simulink model "testing"  (R2023b)
settings: Solver=FixedStepAuto  StartTime=0.0  StopTime=2  FixedStep=0.001  MaxStep=0.02  RelTol=1e-3
undefined symbols (not defined in the file or in its folder): b_t, bt_eq, i_t, Jt_eq, m_t, r_td
libraries: robotcorelib x2
settings Model: Creator=Ferran  LastModifiedBy=Ferran

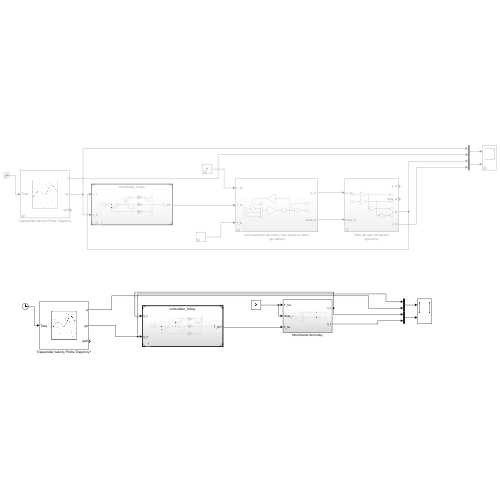
[thumbnail: Simulink's stored preview of the top-level diagram]
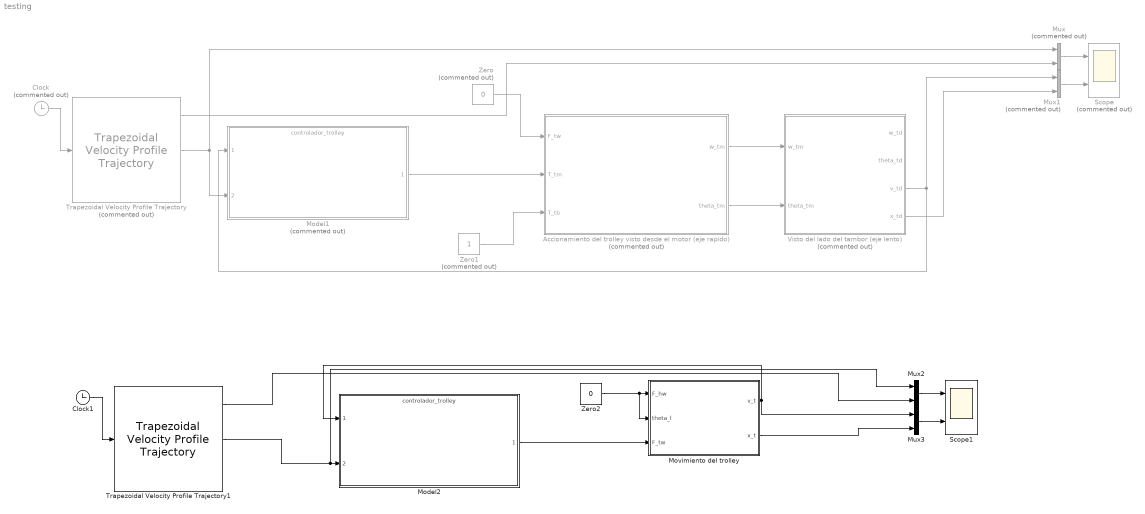
== system testing ==
  Accionamiento del trolley visto desde el motor (eje rapido) : Subsystem  Commented=on
  Clock : Clock  Commented=on
  Clock1 : Clock
  Model1 : ModelReference  Commented=on  ModelNameDialog=controlador_trolley.slx  SimulationMode=Normal  ModelReferenceVersion=2.14
  Model2 : ModelReference  ModelNameDialog=controlador_trolley.slx  SimulationMode=Normal  ModelReferenceVersion=2.15
  Movimiento del trolley : Subsystem
  Mux : Mux  Commented=on  Inputs=2
  Mux1 : Mux  Commented=on  Inputs=2
  Mux2 : Mux  Inputs=2
  Mux3 : Mux  Inputs=2
  Scope : Scope  Commented=on  NumInputPorts=2
  Scope1 : Scope  NumInputPorts=2
  Trapezoidal Velocity Profile Trajectory : robotcorelib/Trapezoidal Velocity Profile Trajectory  Commented=on  WaypointSource=Internal  Waypoints=[0, 1]  NumParams=1  Parameter1=Peak Velocity  Parameter2=End Time  ParameterSource=Internal  PeakVelocity=[ 4 ]  Acceleration=[ 1; 2 ]  EndTime=[ 1]  AccelTime=[ 1; 2 ]  SimulateUsing=Interpreted execution
  Trapezoidal Velocity Profile Trajectory1 : robotcorelib/Trapezoidal Velocity Profile Trajectory  WaypointSource=Internal  Waypoints=[0, 1]  NumParams=1  Parameter1=Peak Velocity  Parameter2=End Time  ParameterSource=Internal  PeakVelocity=[ 4 ]  Acceleration=[ 1; 2 ]  EndTime=[ 1]  AccelTime=[ 1; 2 ]  SimulateUsing=Interpreted execution
  Visto del lado del tambor (eje lento) : Subsystem  Commented=on
  Zero : Constant  Commented=on  Value=0  OutDataTypeStr=Inherit: Inherit via back propagation
  Zero1 : Constant  Commented=on  OutDataTypeStr=Inherit: Inherit via back propagation
  Zero2 : Constant  Value=0  OutDataTypeStr=Inherit: Inherit via back propagation
  wires:
  Zero/1 -> Accionamiento del trolley visto desde el motor (eje rapido)/1(F_tw)
  Model1/1 -> Accionamiento del trolley visto desde el motor (eje rapido)/2(T_tm)
  Zero1/1 -> Accionamiento del trolley visto desde el motor (eje rapido)/3(T_tb)
  Clock/1 -> Trapezoidal Velocity Profile Trajectory/1
  Trapezoidal Velocity Profile Trajectory/2 -> Mux/1, Model1/2
  Trapezoidal Velocity Profile Trajectory/1 -> Mux/2
  Accionamiento del trolley visto desde el motor (eje rapido)/1(w_tm) -> Visto del lado del tambor (eje lento)/1(w_tm)
  Accionamiento del trolley visto desde el motor (eje rapido)/2(theta_tm) -> Visto del lado del tambor (eje lento)/2(theta_tm)
  Visto del lado del tambor (eje lento)/3(v_td) -> Mux1/1, Model1/1
  Visto del lado del tambor (eje lento)/4(x_td) -> Mux1/2
  Mux1/1 -> Scope/2
  Mux/1 -> Scope/1
  Movimiento del trolley/1(v_t) -> Mux3/1, Model2/1
  Model2/1 -> Movimiento del trolley/3(F_tw)
  Clock1/1 -> Trapezoidal Velocity Profile Trajectory1/1
  Zero2/1 -> Movimiento del trolley/2(theta_l), Movimiento del trolley/1(F_hw)
  Movimiento del trolley/2(x_t) -> Mux3/2
  Trapezoidal Velocity Profile Trajectory1/2 -> Mux2/1, Model2/2
  Mux3/1 -> Scope1/2
  Mux2/1 -> Scope1/1
  Trapezoidal Velocity Profile Trajectory1/1 -> Mux2/2

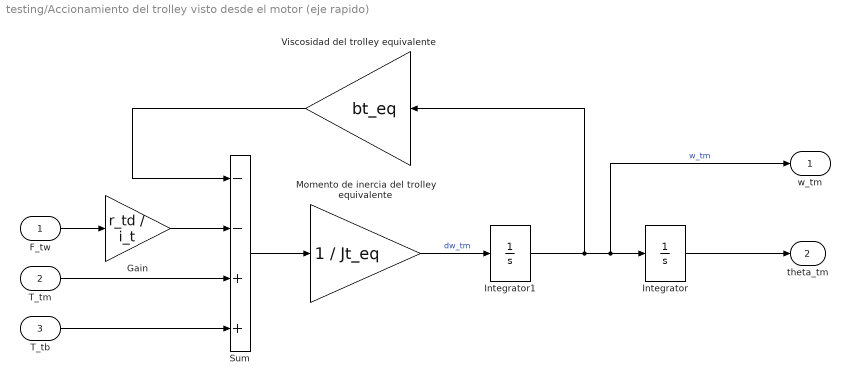
== system testing/Accionamiento del trolley visto desde el motor (eje rapido) ==
  F_tw : Inport
  T_tm : Inport  Port=2
  T_tb : Inport  Port=3
  Gain : Gain  Gain=r_td / i_t
  Integrator : Integrator
  Integrator1 : Integrator
  Momento de inercia del trolley equivalente : Gain  Gain=1 / Jt_eq
  Sum : Sum  Inputs=--++
  Viscosidad del trolley equivalente : Gain  Gain=bt_eq
  w_tm : Outport
  theta_tm : Outport  Port=2
  wires:
  Gain/1 -> Sum/2
  Integrator/1 -> theta_tm/1
  Sum/1 -> Momento de inercia del trolley equivalente/1
  Integrator1/1 -> Viscosidad del trolley equivalente/1, w_tm/1, Integrator/1  "w_tm"
  Viscosidad del trolley equivalente/1 -> Sum/1
  Momento de inercia del trolley equivalente/1 -> Integrator1/1  "dw_tm"
  F_tw/1 -> Gain/1
  T_tb/1 -> Sum/4
  T_tm/1 -> Sum/3

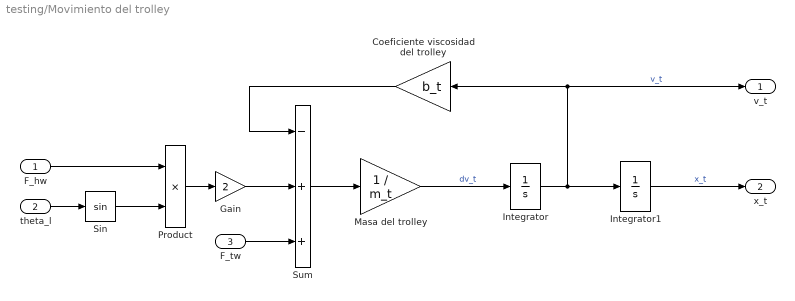
== system testing/Movimiento del trolley ==
  F_hw : Inport
  theta_l : Inport  Port=2
  F_tw : Inport  Port=3
  Coeficiente viscosidad del trolley : Gain  Gain=b_t
  Gain : Gain  Gain=2
  Integrator : Integrator
  Integrator1 : Integrator
  Masa del trolley : Gain  Gain=1 / m_t
  Product : Product
  Sin : Trigonometry
  Sum : Sum  Inputs=-++
  v_t : Outport
  x_t : Outport  Port=2
  wires:
  Sin/1 -> Product/2
  F_tw/1 -> Sum/3
  Integrator/1 -> v_t/1, Coeficiente viscosidad del trolley/1, Integrator1/1  "v_t"
  F_hw/1 -> Product/1
  Integrator1/1 -> x_t/1  "x_t"
  Product/1 -> Gain/1
  Sum/1 -> Masa del trolley/1
  theta_l/1 -> Sin/1
  Masa del trolley/1 -> Integrator/1  "dv_t"
  Gain/1 -> Sum/2
  Coeficiente viscosidad del trolley/1 -> Sum/1

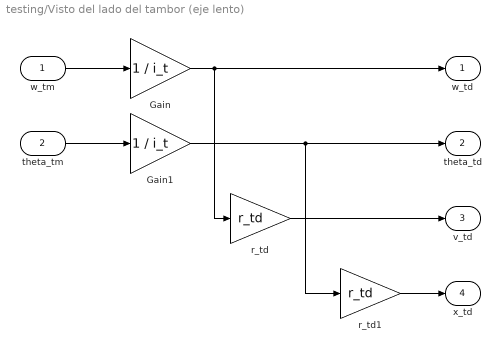
== system testing/Visto del lado del tambor (eje lento) ==
  w_tm : Inport
  theta_tm : Inport  Port=2
  Gain : Gain  Gain=1 / i_t
  Gain1 : Gain  Gain=1 / i_t
  r_td : Gain  Gain=r_td
  r_td1 : Gain  Gain=r_td
  w_td : Outport
  theta_td : Outport  Port=2
  v_td : Outport  Port=3
  x_td : Outport  Port=4
  wires:
  Gain1/1 -> r_td1/1, theta_td/1
  Gain/1 -> w_td/1, r_td/1
  w_tm/1 -> Gain/1
  theta_tm/1 -> Gain1/1
  r_td/1 -> v_td/1
  r_td1/1 -> x_td/1
